simulink model "SrmAmLinearApcZhw3a3tst"  (R2013b)
settings: Solver=ode45  StartTime=0.0  StopTime=0.05  MaxStep=5e-5  RelTol=1e-3
InitFcn:
  | theta0=30*2*pi/360;
  | ks=1.22;
  | is=2;
  | lu=0.016;
  | rs=1.5;
  | lux=1;
  | j=0.01;
settings Model: Creator=mamingkai  LastModifiedBy=Think79

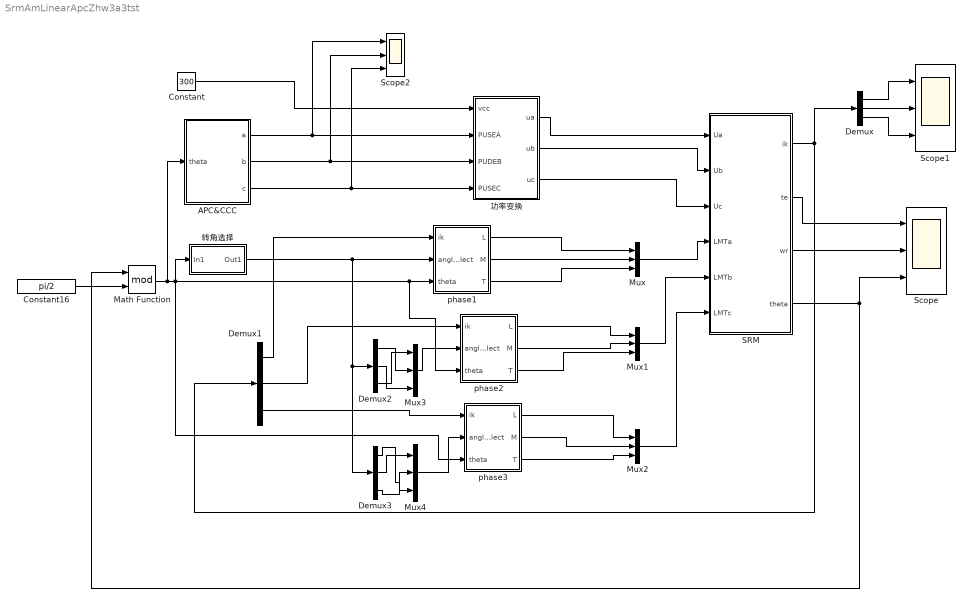
== system SrmAmLinearApcZhw3a3tst ==
  APC&CCC : Subsystem
  Constant : Constant  Value=300
  Constant16 : Constant  Value=pi/2
  Demux{,1..3} (4 alike) : Demux  Outputs=3
  Math Function : Math  Operator=mod  SaturateOnIntegerOverflow=on
  Mux{,1..4} (5 alike) : Mux  Inputs=3
  SRM : Subsystem
  Scope : Scope  NumInputPorts=3
      settings: TimeRange=0.2  YMin=-100~-10~-1  YMax=200~30~3
  Scope1 : Scope  NumInputPorts=3
      settings: YMin=-5~-5~-5  YMax=5~5~5  SaveName=ScopeData6
  Scope2 : Scope  NumInputPorts=3
      settings: TimeRange=0.2  YMin=-100~-10~-1  YMax=200~30~3  SaveName=ScopeData27
  phase1 : Subsystem
  phase2 : Subsystem
  phase3 : Subsystem
  功率变换 : Subsystem
  转角选择 : Subsystem
  wires:
  APC&CCC/1(a) -> 功率变换/2(PUSEA), Scope2/1
  APC&CCC/2(b) -> 功率变换/3(PUDEB), Scope2/2
  APC&CCC/3(c) -> 功率变换/4(PUSEC), Scope2/3
  Constant/1 -> 功率变换/1(vcc)
  功率变换/1(ua) -> SRM/1(Ua)
  功率变换/2(ub) -> SRM/2(Ub)
  功率变换/3(uc) -> SRM/3(Uc)
  SRM/3(wr) -> Scope/2
  SRM/4(theta) -> Math Function/1, Scope/3
  SRM/2(te) -> Scope/1
  Demux/1 -> Scope1/1
  Demux/2 -> Scope1/2
  Demux/3 -> Scope1/3
  Mux/1 -> SRM/4(LMTa)
  SRM/1(ik) -> Demux1/1, Demux/1
  Demux1/1 -> phase1/1(ik)
  Demux1/2 -> phase2/1(ik)
  Demux1/3 -> phase3/1(ik)
  Mux1/1 -> SRM/5(LMTb)
  Mux2/1 -> SRM/6(LMTc)
  Mux3/1 -> phase2/2("angleselect ")
  转角选择/1(Out1) -> Demux3/1, Demux2/1, phase1/2("angleselect ")
  Mux4/1 -> phase3/2("angleselect ")
  Demux3/1 -> Mux4/3
  Demux3/2 -> Mux4/1
  Demux3/3 -> Mux4/2
  Demux2/1 -> Mux3/2
  Demux2/2 -> Mux3/3
  Demux2/3 -> Mux3/1
  phase1/1("L ") -> Mux/1
  phase1/2(M) -> Mux/2
  phase1/3(T) -> Mux/3
  phase2/1("L ") -> Mux1/1
  phase2/2(M) -> Mux1/2
  phase2/3(T) -> Mux1/3
  phase3/1("L ") -> Mux2/1
  phase3/2(M) -> Mux2/2
  phase3/3(T) -> Mux2/3
  Constant16/1 -> Math Function/2
  Math Function/1 -> APC&CCC/1(theta), phase3/3(theta), 转角选择/1(In1), phase2/3(theta), phase1/3(theta)

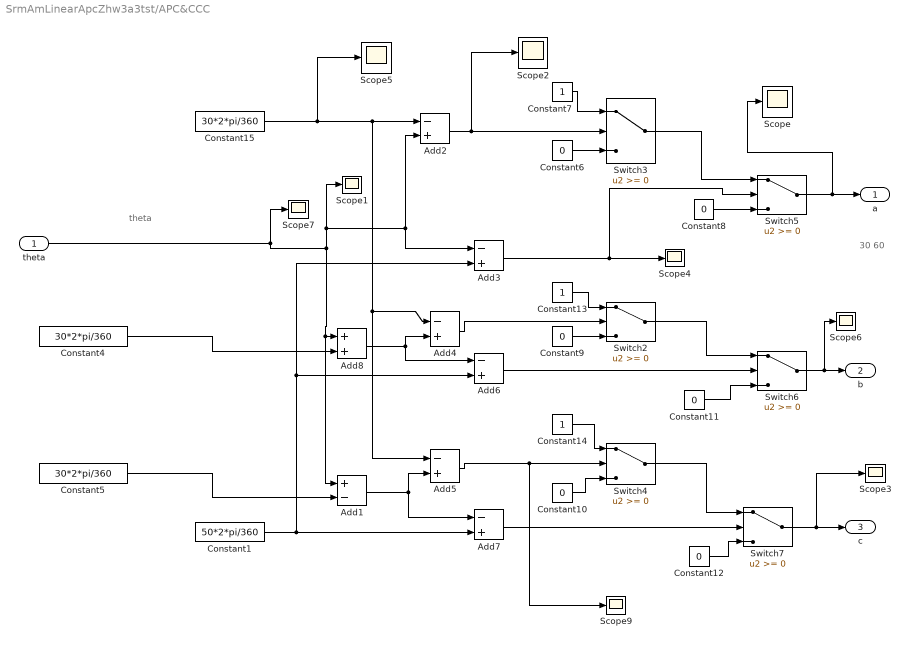
== system SrmAmLinearApcZhw3a3tst/APC&CCC ==
  note: 30 60
  note: theta
  theta : Inport
  Add1 : Sum  Inputs=+-
  Add{2..7} (6 alike) : Sum  Inputs=-+
  Add8 : Sum
  Constant1 : Constant  Value=50*2*pi/360
  Constant{6,8..12} (6 alike) : Constant  Value=0
  Constant13 : Constant
  Constant14 : Constant
  Constant15 : Constant  Value=30*2*pi/360
  Constant4 : Constant  Value=30*2*pi/360
  Constant5 : Constant  Value=30*2*pi/360
  Constant7 : Constant
  Scope{,1..7,9} (9 alike) : Scope
      Scope settings: TimeRange=2  YMin=-1  YMax=1  SaveName=ScopeData3
      Scope1 settings: SaveName=ScopeData5
      Scope2 settings: TimeRange=2  YMin=-1  YMax=1  SaveName=ScopeData7
      Scope3 settings: SaveName=ScopeData8
      Scope4 settings: SaveName=ScopeData9
      Scope5 settings: TimeRange=2  YMin=-1  YMax=1  SaveName=ScopeData10
      Scope6 settings: SaveName=ScopeData11
      Scope7 settings: YMin=0.2  YMax=0.85  SaveName=ScopeData19
      Scope9 settings: YMin=0.2  YMax=0.85  SaveName=ScopeData21
  Switch{2..7} (6 alike) : Switch
  a : Outport
  b : Outport  Port=2
  c : Outport  Port=3
  wires:
  Switch5/1 -> Scope/1, a/1
  Constant1/1 -> Add3/2, Add6/2, Add7/2
  Constant15/1 -> Scope5/1, Add5/1, Add4/1, Add2/1
  Add3/1 -> Switch5/2, Scope4/1
  Add6/1 -> Switch6/2
  Add7/1 -> Switch7/2
  Constant6/1 -> Switch3/3
  Switch3/1 -> Switch5/1
  Switch2/1 -> Switch6/1
  Switch4/1 -> Switch7/1
  Switch6/1 -> Scope6/1, b/1
  Switch7/1 -> Scope3/1, c/1
  Add2/1 -> Scope2/1, Switch3/2
  Constant12/1 -> Switch7/3
  Constant11/1 -> Switch6/3
  Constant10/1 -> Switch4/3
  Constant9/1 -> Switch2/3
  Constant8/1 -> Switch5/3
  Constant7/1 -> Switch3/1
  Constant13/1 -> Switch2/1
  Constant14/1 -> Switch4/1
  Add5/1 -> Scope9/1, Switch4/2
  Add4/1 -> Switch2/2
  theta/1 -> Scope1/1, Add3/1, Add2/2, Add8/1, Add1/1, Scope7/1
  Constant5/1 -> Add1/2
  Add1/1 -> Add5/2, Add7/1
  Constant4/1 -> Add8/2
  Add8/1 -> Add6/1, Add4/2

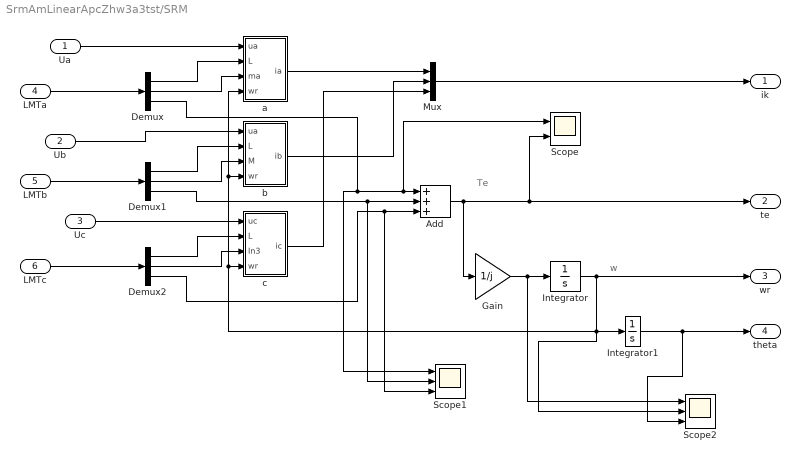
== system SrmAmLinearApcZhw3a3tst/SRM ==
  note: w
  note: Te
  Ua : Inport
  Ub : Inport  Port=2
  Uc : Inport  Port=3
  LMTa : Inport  Port=4
  LMTb : Inport  Port=5
  LMTc : Inport  Port=6
  Add : Sum  Inputs=+++
  Demux : Demux  Outputs=3
  Demux1 : Demux  Outputs=3
  Demux2 : Demux  Outputs=3
  Gain : Gain  Gain=1/j
  Integrator : Integrator
  Integrator1 : Integrator  InitialCondition=5*2*pi/360
  Mux : Mux  Inputs=3
  Scope : Scope  NumInputPorts=2
      settings: YMin=-5~-5  YMax=5~5
  Scope1 : Scope  NumInputPorts=3
      settings: YMin=-5~-5~-5  YMax=5~5~5  SaveName=ScopeData22
  Scope2 : Scope  NumInputPorts=3
      settings: YMin=-5~-5~-5  YMax=5~5~5  SaveName=ScopeData29
  a : Subsystem
  b : Subsystem
  c : Subsystem
  ik : Outport
  te : Outport  Port=2
  wr : Outport  Port=3
  theta : Outport  Port=4
  wires:
  LMTa/1 -> Demux/1
  Demux/1 -> a/2("L ")
  Demux/2 -> a/3(ma)
  Demux/3 -> Scope/1, Add/1, Scope1/1
  Ub/1 -> b/1(ua)
  Demux1/1 -> b/2(L)
  Demux1/2 -> b/3(M)
  Uc/1 -> c/1("uc ")
  LMTc/1 -> Demux2/1
  LMTb/1 -> Demux1/1
  Demux2/1 -> c/2(L)
  Demux2/2 -> c/3(In3)
  Demux2/3 -> Add/3, Scope1/3
  Integrator/1 -> wr/1, Scope2/2, c/4(wr), b/4("wr "), a/4(wr), Integrator1/1
  a/1(ia) -> Mux/1
  b/1("ib ") -> Mux/2
  c/1(ic) -> Mux/3
  Mux/1 -> ik/1
  Add/1 -> Gain/1, te/1, Scope/2
  Gain/1 -> Scope2/1, Integrator/1
  Ua/1 -> a/1(ua)
  Demux1/3 -> Add/2, Scope1/2
  Integrator1/1 -> Scope2/3, theta/1

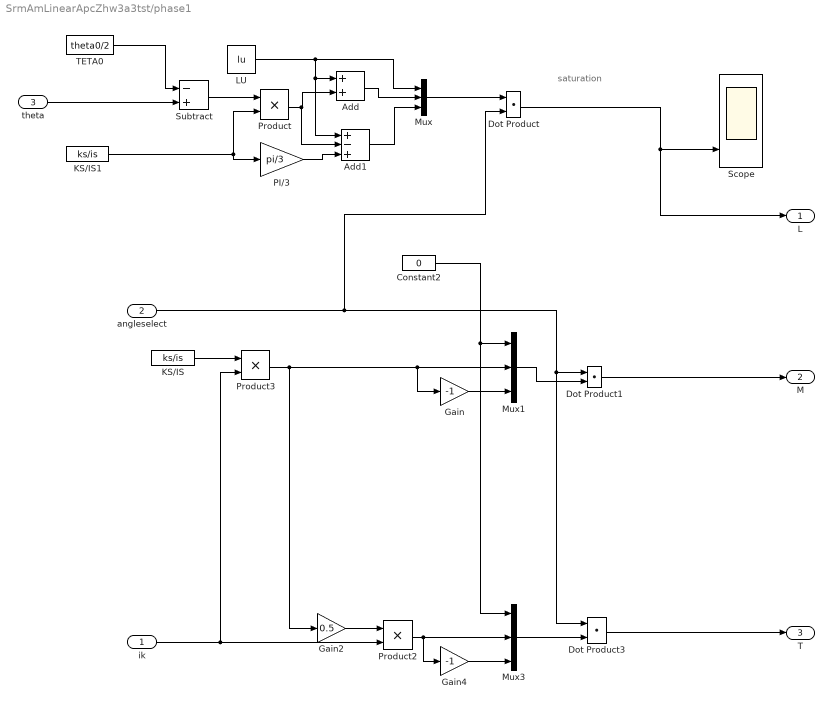
== system SrmAmLinearApcZhw3a3tst/phase1 ==
  note: saturation
  ik : Inport
  "angleselect " : Inport  Port=2
  theta : Inport  Port=3
  Add : Sum
  Add1 : Sum  Inputs=+-+
  Constant2 : Constant  Value=0
  Dot Product : DotProduct  InputSameDT=on  OutDataTypeStr=Inherit: Inherit via internal rule
  Dot Product1 : DotProduct  InputSameDT=on  OutDataTypeStr=Inherit: Inherit via internal rule
  Dot Product3 : DotProduct  InputSameDT=on  OutDataTypeStr=Inherit: Inherit via internal rule
  Gain : Gain  Gain=-1
  Gain2 : Gain  Gain=0.5
  Gain4 : Gain  Gain=-1
  KS/IS : Constant  Value=ks/is
  KS/IS1 : Constant  Value=ks/is
  LU : Constant  Value=lu
  Mux : Mux  Inputs=3
  Mux1 : Mux  Inputs=3
  Mux3 : Mux  Inputs=3
  PI/3 : Gain  Gain=pi/3
  Product : Product
  Product2 : Product
  Product3 : Product
  Scope : Scope  NumInputPorts=3
      settings: TimeRange=0.2  YMin=-100~-10~-1  YMax=200~30~3  SaveName=ScopeData4
  Subtract : Sum  Inputs=-+
  TETA0 : Constant  Value=theta0/2
  "L " : Outport
  M : Outport  Port=2
  T : Outport  Port=3
  wires:
  Dot Product/1 -> "L "/1, Scope/3
  KS/IS/1 -> Product3/1
  ik/1 -> Product3/2, Product2/2
  Constant2/1 -> Mux3/1, Mux1/1
  Mux3/1 -> Dot Product3/2
  Mux1/1 -> Dot Product1/2
  Product3/1 -> Gain/1, Mux1/2, Gain2/1
  Gain/1 -> Mux1/3
  Gain2/1 -> Product2/1
  Dot Product1/1 -> M/1
  Dot Product3/1 -> T/1
  Product2/1 -> Gain4/1, Mux3/2
  Gain4/1 -> Mux3/3
  theta/1 -> Subtract/2
  TETA0/1 -> Subtract/1
  Subtract/1 -> Product/1
  KS/IS1/1 -> PI/3/1, Product/2
  LU/1 -> Mux/1, Add1/1, Add/1
  Product/1 -> Add1/2, Add/2
  PI/3/1 -> Add1/3
  Add/1 -> Mux/2
  Add1/1 -> Mux/3
  Mux/1 -> Dot Product/1
  "angleselect "/1 -> Dot Product/2, Dot Product3/1, Dot Product1/1

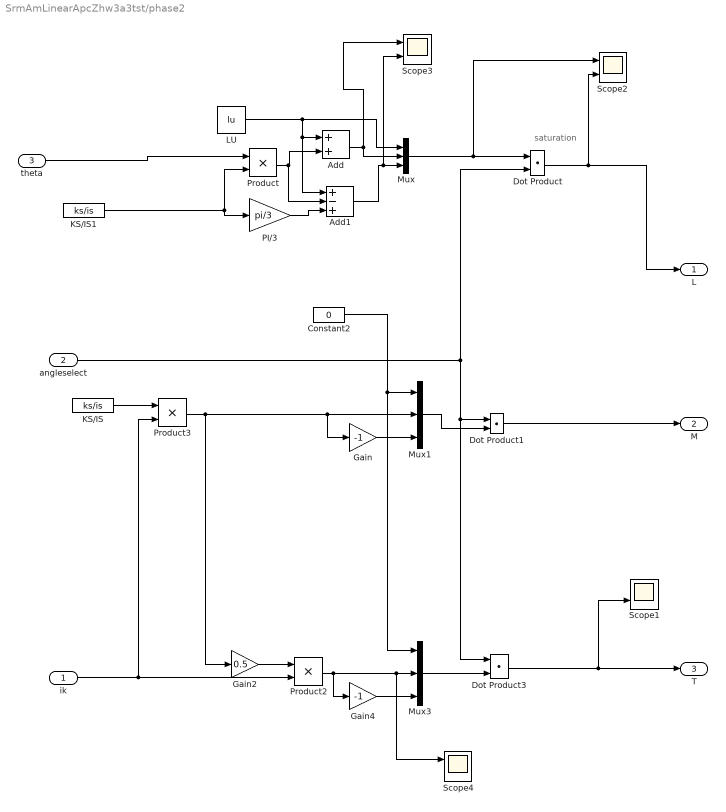
== system SrmAmLinearApcZhw3a3tst/phase2 ==
  note: saturation
  ik : Inport
  "angleselect " : Inport  Port=2
  theta : Inport  Port=3
  Add : Sum
  Add1 : Sum  Inputs=+-+
  Constant2 : Constant  Value=0
  Dot Product : DotProduct  InputSameDT=on  OutDataTypeStr=Inherit: Inherit via internal rule
  Dot Product1 : DotProduct  InputSameDT=on  OutDataTypeStr=Inherit: Inherit via internal rule
  Dot Product3 : DotProduct  InputSameDT=on  OutDataTypeStr=Inherit: Inherit via internal rule
  Gain : Gain  Gain=-1
  Gain2 : Gain  Gain=0.5
  Gain4 : Gain  Gain=-1
  KS/IS : Constant  Value=ks/is
  KS/IS1 : Constant  Value=ks/is
  LU : Constant  Value=lu
  Mux : Mux  Inputs=3
  Mux1 : Mux  Inputs=3
  Mux3 : Mux  Inputs=3
  PI/3 : Gain  Gain=pi/3
  Product : Product
  Product2 : Product
  Product3 : Product
  Scope{1..4} (4 alike) : Scope  NumInputPorts=2
      Scope1 settings: YMin=-5~-5  YMax=5~5  SaveName=ScopeData24
      Scope2 settings: YMin=-5~-5  YMax=5~5  SaveName=ScopeData15
      Scope3 settings: YMin=-5~-5  YMax=5~5  SaveName=ScopeData30
      Scope4 settings: YMin=-5~-5  YMax=5~5  SaveName=ScopeData20
  "L " : Outport
  M : Outport  Port=2
  T : Outport  Port=3
  wires:
  Gain4/1 -> Mux3/3
  Product2/1 -> Scope4/1, Mux3/2, Gain4/1
  Dot Product3/1 -> Scope1/2, T/1
  Dot Product1/1 -> M/1
  Gain2/1 -> Product2/1
  Gain/1 -> Mux1/3
  Product3/1 -> Gain2/1, Mux1/2, Gain/1
  Mux1/1 -> Dot Product1/2
  Mux3/1 -> Dot Product3/2
  Constant2/1 -> Mux1/1, Mux3/1
  ik/1 -> Product2/2, Product3/2
  KS/IS/1 -> Product3/1
  Dot Product/1 -> Scope2/2, "L "/1
  theta/1 -> Product/1
  KS/IS1/1 -> PI/3/1, Product/2
  LU/1 -> Mux/1, Add1/1, Add/1
  Product/1 -> Add1/2, Add/2
  PI/3/1 -> Add1/3
  Add/1 -> Mux/2, Scope3/1
  Add1/1 -> Scope3/2, Mux/3
  Mux/1 -> Scope2/1, Dot Product/1
  "angleselect "/1 -> Dot Product1/1, Dot Product3/1, Dot Product/2

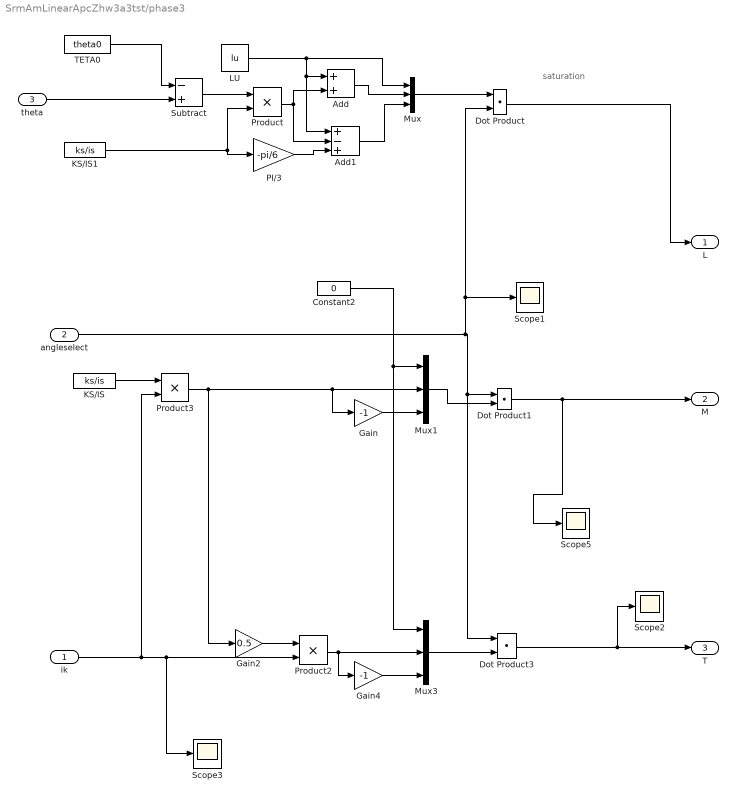
== system SrmAmLinearApcZhw3a3tst/phase3 ==
  note: saturation
  ik : Inport
  "angleselect " : Inport  Port=2
  theta : Inport  Port=3
  Add : Sum
  Add1 : Sum  Inputs=+-+
  Constant2 : Constant  Value=0
  Dot Product : DotProduct  InputSameDT=on  OutDataTypeStr=Inherit: Inherit via internal rule
  Dot Product1 : DotProduct  InputSameDT=on  OutDataTypeStr=Inherit: Inherit via internal rule
  Dot Product3 : DotProduct  InputSameDT=on  OutDataTypeStr=Inherit: Inherit via internal rule
  Gain : Gain  Gain=-1
  Gain2 : Gain  Gain=0.5
  Gain4 : Gain  Gain=-1
  KS/IS : Constant  Value=ks/is
  KS/IS1 : Constant  Value=ks/is
  LU : Constant  Value=lu
  Mux : Mux  Inputs=3
  Mux1 : Mux  Inputs=3
  Mux3 : Mux  Inputs=3
  PI/3 : Gain  Gain=-pi/6
  Product : Product
  Product2 : Product
  Product3 : Product
  Scope{1..3,5} (4 alike) : Scope
      Scope1 settings: TimeRange=2  YMin=-1  YMax=1  SaveName=ScopeData17
      Scope2 settings: TimeRange=2  YMin=-1  YMax=1  SaveName=ScopeData23
      Scope3 settings: TimeRange=2  YMin=-1  YMax=1  SaveName=ScopeData25
      Scope5 settings: TimeRange=2  YMin=-1  YMax=1  SaveName=ScopeData16
  Subtract : Sum  Inputs=-+
  TETA0 : Constant  Value=theta0
  "L " : Outport
  M : Outport  Port=2
  T : Outport  Port=3
  wires:
  Dot Product/1 -> "L "/1
  KS/IS/1 -> Product3/1
  ik/1 -> Product3/2, Scope3/1, Product2/2
  Constant2/1 -> Mux3/1, Mux1/1
  Mux3/1 -> Dot Product3/2
  Mux1/1 -> Dot Product1/2
  Product3/1 -> Gain/1, Mux1/2, Gain2/1
  Gain/1 -> Mux1/3
  Gain2/1 -> Product2/1
  Dot Product1/1 -> Scope5/1, M/1
  Dot Product3/1 -> Scope2/1, T/1
  Product2/1 -> Gain4/1, Mux3/2
  Gain4/1 -> Mux3/3
  theta/1 -> Subtract/2
  TETA0/1 -> Subtract/1
  Subtract/1 -> Product/1
  KS/IS1/1 -> PI/3/1, Product/2
  LU/1 -> Mux/1, Add1/1, Add/1
  Product/1 -> Add1/2, Add/2
  PI/3/1 -> Add1/3
  Add/1 -> Mux/2
  Add1/1 -> Mux/3
  Mux/1 -> Dot Product/1
  "angleselect "/1 -> Dot Product/2, Scope1/1, Dot Product3/1, Dot Product1/1

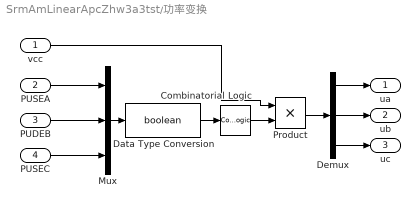
== system SrmAmLinearApcZhw3a3tst/功率变换 ==
  vcc : Inport
  PUSEA : Inport  Port=2
  PUDEB : Inport  Port=3
  PUSEC : Inport  Port=4
  Combinatorial Logic : CombinatorialLogic  TruthTable=[0 0 0 ;0 0 1;0 1 0;0 1 1;1 0 0;1 0 1;1 1 0;1 1 1]
  Data Type Conversion : DataTypeConversion  OutDataTypeStr=boolean
  Demux : Demux  Outputs=3
  Mux : Mux  Inputs=3
  Product : Product
  ua : Outport
  ub : Outport  Port=2
  uc : Outport  Port=3
  wires:
  PUSEA/1 -> Mux/1
  Demux/1 -> ua/1
  Product/1 -> Demux/1
  Demux/2 -> ub/1
  Demux/3 -> uc/1
  PUDEB/1 -> Mux/2
  PUSEC/1 -> Mux/3
  Combinatorial Logic/1 -> Product/2
  vcc/1 -> Product/1
  Mux/1 -> Data Type Conversion/1
  Data Type Conversion/1 -> Combinatorial Logic/1

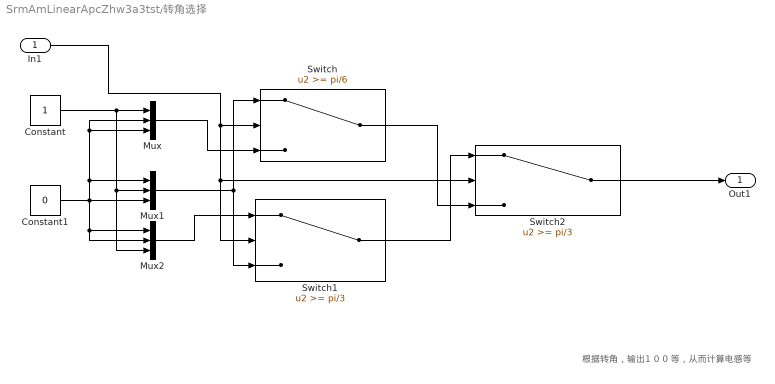
== system SrmAmLinearApcZhw3a3tst/转角选择 ==
  note: 根据转角，输出1 0 0 等，从而计算电感等
  In1 : Inport
  Constant : Constant
  Constant1 : Constant  Value=0
  Mux : Mux  Inputs=3
  Mux1 : Mux  Inputs=3
  Mux2 : Mux  Inputs=3
  Switch : Switch  Threshold=pi/6
  Switch1 : Switch  Threshold=pi/3
  Switch2 : Switch  Threshold=pi/3
  Out1 : Outport
  wires:
  Constant/1 -> Mux2/3, Mux1/2, Mux/1
  Mux/1 -> Switch/3
  Constant1/1 -> Mux/3, Mux/2, Mux1/1, Mux2/2, Mux2/1, Mux1/3
  Mux1/1 -> Switch1/3, Switch/1
  Mux2/1 -> Switch1/1
  In1/1 -> Switch2/2, Switch1/2, Switch/2
  Switch/1 -> Switch2/3
  Switch1/1 -> Switch2/1
  Switch2/1 -> Out1/1

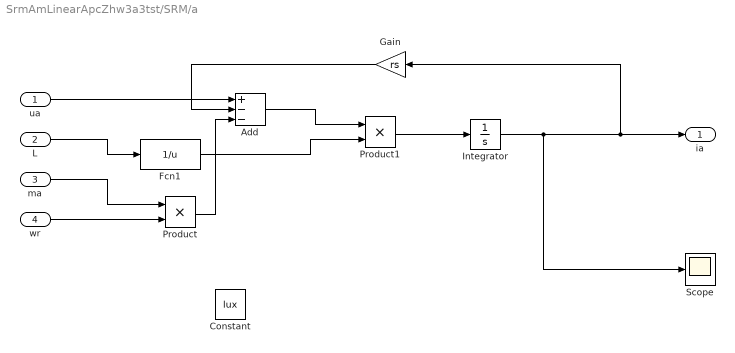
== system SrmAmLinearApcZhw3a3tst/SRM/a ==
  ua : Inport
  "L " : Inport  Port=2
  ma : Inport  Port=3
  wr : Inport  Port=4
  Add : Sum  Inputs=+--
  Constant : Constant  Value=lux
  Fcn1 : Fcn  Expr=1/u
  Gain : Gain  Gain=rs
  Integrator : Integrator
  Product : Product
  Product1 : Product
  Scope : Scope
      settings: SaveName=ScopeData2
  ia : Outport
  wires:
  wr/1 -> Product/2
  Integrator/1 -> Scope/1, Gain/1, ia/1
  ma/1 -> Product/1
  ua/1 -> Add/1
  Gain/1 -> Add/2
  Product/1 -> Add/3
  Add/1 -> Product1/1
  Product1/1 -> Integrator/1
  "L "/1 -> Fcn1/1
  Fcn1/1 -> Product1/2

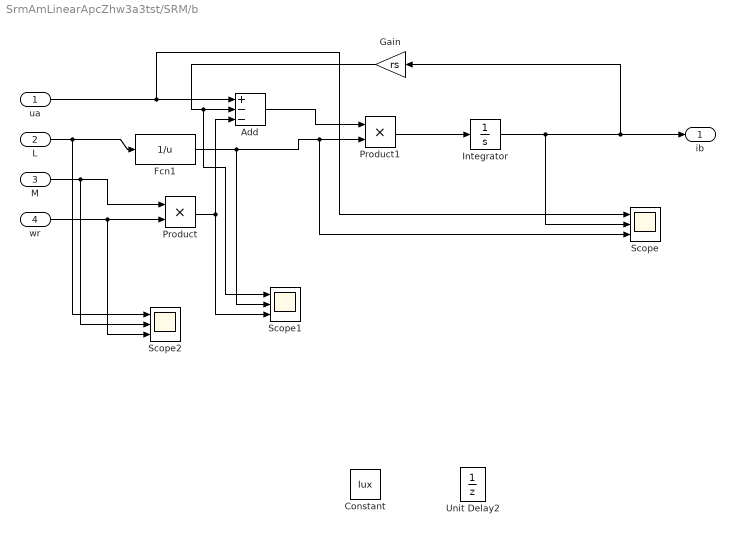
== system SrmAmLinearApcZhw3a3tst/SRM/b ==
  ua : Inport
  L : Inport  Port=2
  M : Inport  Port=3
  "wr " : Inport  Port=4
  Add : Sum  Inputs=+--
  Constant : Constant  Value=lux
  Fcn1 : Fcn  Expr=1/u
  Gain : Gain  Gain=rs
  Integrator : Integrator
  Product : Product
  Product1 : Product
  Scope : Scope  NumInputPorts=3
      settings: YMin=-5~-5~-5  YMax=5~5~5  SaveName=ScopeData18
  Scope1 : Scope  NumInputPorts=3
      settings: YMin=-5~-5~-5  YMax=5~5~5  SaveName=ScopeData28
  Scope2 : Scope  NumInputPorts=3
      settings: YMin=-5~-5~-5  YMax=5~5~5  SaveName=ScopeData31
  Unit Delay2 : UnitDelay  SampleTime=-1
  "ib " : Outport
  wires:
  "wr "/1 -> Scope2/3, Product/2
  M/1 -> Scope2/2, Product/1
  ua/1 -> Scope/1, Add/1
  Gain/1 -> Scope1/1, Add/2
  Product/1 -> Add/3, Scope1/3
  Add/1 -> Product1/1
  Product1/1 -> Integrator/1
  Integrator/1 -> Scope/2, Gain/1, "ib "/1
  L/1 -> Scope2/1, Fcn1/1
  Fcn1/1 -> Scope1/2, Scope/3, Product1/2

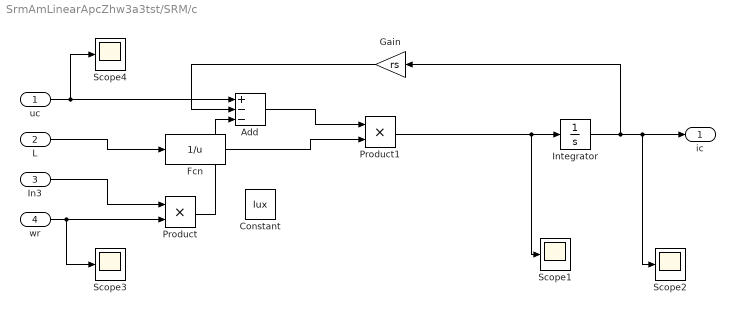
== system SrmAmLinearApcZhw3a3tst/SRM/c ==
  "uc " : Inport
  L : Inport  Port=2
  In3 : Inport  Port=3
  wr : Inport  Port=4
  Add : Sum  Inputs=+--
  Constant : Constant  Value=lux
  Fcn : Fcn  Expr=1/u
  Gain : Gain  Gain=rs
  Integrator : Integrator
  Product : Product
  Product1 : Product
  Scope{1..4} (4 alike) : Scope
      Scope1 settings: TimeRange=2  YMin=-1  YMax=1  SaveName=ScopeData13
      Scope2 settings: TimeRange=2  YMin=-1  YMax=1  SaveName=ScopeData12
      Scope3 settings: TimeRange=2  YMin=-1  YMax=1  SaveName=ScopeData14
      Scope4 settings: TimeRange=2  YMin=-1  YMax=1  SaveName=ScopeData26
  ic : Outport
  wires:
  wr/1 -> Scope3/1, Product/2
  In3/1 -> Product/1
  "uc "/1 -> Scope4/1, Add/1
  Gain/1 -> Add/2
  Product/1 -> Add/3
  Add/1 -> Product1/1
  Integrator/1 -> Gain/1, Scope2/1, ic/1
  L/1 -> Fcn/1
  Product1/1 -> Scope1/1, Integrator/1
  Fcn/1 -> Product1/2
